simulink model "vehicleHVAC"  (R2016a)
settings: Solver=VariableStepAuto  SolverMode=SingleTasking  StartTime=0.0  StopTime=2000  RelTol=1e-3
PreLoadFcn:
  | T_init = 25; % degC
  | RH_init = 0.5;
  | p_env = 101.325; % kPa
  | 
  | T_coolant = 90; % degC
  | C_coolant = 0.7; % kW/K
  | T_refrigerant = 4; % degC
  | 
  | cabin_volume = 3; % m^3
  | duct_area = 0.015; % m^2
StartFcn:
  | if strcmp(get_param([bdroot, '/System Inputs'], 'OverrideUsingVariant'), 'Manual')
  | 
  |     if exist('h1_vehicleHVAC', 'var') && isgraphics(h1_vehicleHVAC, 'figure')
  |         h1_vehicleHVAC.prepManualInput()
  |     end
  | 
  |     clear updatePsychrometricChart
  |     listener_vehicleHVAC = add_exec_event_listener( ...
  |         [bdroot '/Cabin/Cabin Sensors/Cabin Outputs'], ...
  |         'PostOutputs', ...
  |         @updatePsychrometricChart);
  | 
  | else
  | 
  |     clear listener_vehicleHVAC
  | 
  | end
StopFcn:
  | clear listener_vehicleHVAC
undefined symbols (not defined in the file or in its folder): sigbuilder_block
libraries: fl_lib x26, nesl_utility x22, HVAC_lib x16
CloseFcn:
  | try, close(h1_vehicleHVAC), end
  | clear h1_vehicleHVAC
  | 
  | clear simlog_vehicleHVAC tout
  | clear T_init RH_init p_env T_coolant C_coolant T_refrigerant cabin_volume duct_area
Description:
  | Vehicle HVAC System
  | 
  | Copyright 2017 The MathWorks, Inc.
settings Model: Creator=leong  LastModifiedBy=leong
settings SolverCC: MaxConsecutiveMinStep=2
settings DataIOCC: LimitDataPoints=on  MaxDataPoints=10000
settings DebuggingCC: SFUnexpectedBacktrackingDiag=error  SFNoUnconditionalDefaultTransitionDiag=error
settings GRTTargetCC: TargetLangStandard=C99 (ISO)  GeneratePreprocessorConditionals=Use local settings
settings ConfigComp: CovMetricSettings=dwe  CovHtmlReporting=off  CovSaveCumulativeToWorkspaceVar=off  CovSaveSingleToWorkspaceVar=off  CovExternalEMLEnable=on
settings SimscapeCC: SimscapeLogType=all  SimscapeLogSimulationStatistics=on  SimscapeLogName=simlog_vehicleHVAC  SimscapeLogDataHistory=10000

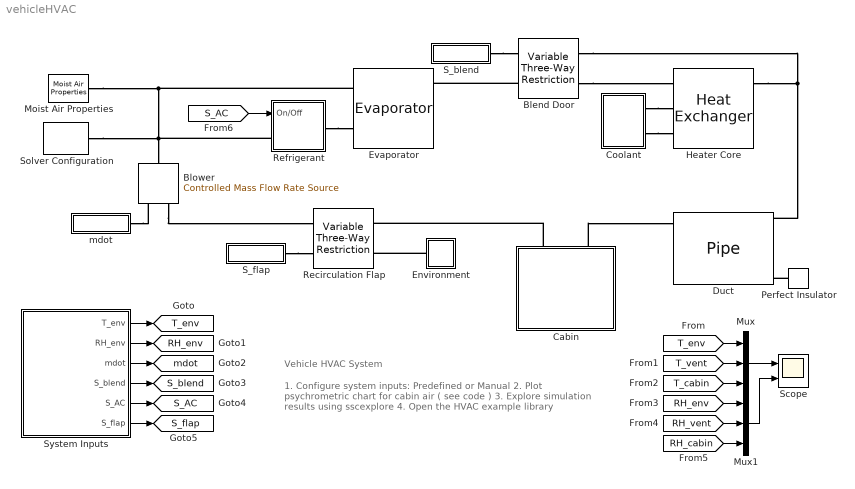
== system vehicleHVAC ==
  note: Vehicle HVAC System
  note: 1. Configure system inputs: Predefined or Manual
      | 2. Plot psychrometric chart for cabin air ( see code )
      | 3. Explore simulation results using sscexplore
      | 4. Open the HVAC example library
  Blend Door : HVAC_lib/Variable Three-Way Restriction  min_area=1e-10 m^2  max_area=0.9 * duct_area m^2  area=duct_area m^2  Cd=0.8  B_lam=0.999
  Blower : HVAC_lib/Controlled Mass Flow Rate Source  flow_area_A=0.01 m^2  flow_area_B=0.01 m^2  area_A=duct_area m^2  area_B=duct_area m^2  mdot_A_specify=off  mdot_A_priority=None  mdot_A=1e-6 kg/s  mdot_B_specify=off  mdot_B_priority=None  mdot_B=1e-6 kg/s  Phi_A_specify=off  Phi_A_priority=None  Phi_A=0 kW  Phi_B_specify=off  Phi_B_priority=None  Phi_B=0 kW  mdot_w_A_specify=off  mdot_w_A_priority=None  mdot_w_A=0 g/s  mdot_w_B_specify=off  mdot_w_B_priority=None  mdot_w_B=0 g/s  h_out_specify=off  h_out_priority=None  h_out=420 kJ/kg  x_w_out_specify=off  x_w_out_priority=None  x_w_out=0.007  power_specify=off  power_priority=None  power=0 kW
  Cabin : Subsystem  Tag=PublishSubsystem  mask{N_occupant=1, W_occupant=0.04, T_occupant=30, Q_occupant=70}
      mask prompts: N_occupant "Number of occupants"; W_occupant "Moisture gain per occupant (g/s)"; T_occupant "Temperature of added moisture (degC)"; Q_occupant "Sensible heat per occupant (W)"
  Coolant : Subsystem
  Duct : HVAC_lib/Pipe  flow_area_A=0.01 m^2  flow_area_B=0.01 m^2  length=1 m  area=duct_area m^2  Dh=sqrt(duct_area) m  length_add=0 m  roughness=15e-6 m  Re_lam=2000  Re_tur=4000  shape_factor=64  Nu_lam=3.66  time_constant=1e-3 s  mdot_A_specify=off  mdot_A_priority=None  mdot_A=1e-6 kg/s  mdot_B_specify=off  mdot_B_priority=None  mdot_B=1e-6 kg/s  Phi_A_specify=off  Phi_A_priority=None  Phi_A=0 kW  Phi_B_specify=off  Phi_B_priority=None  Phi_B=0 kW  mdot_w_A_specify=off  mdot_w_A_priority=None  mdot_w_A=0 g/s  mdot_w_B_specify=off  mdot_w_B_priority=None  mdot_w_B=0 g/s  h_out_specify=off  h_out_priority=None  h_out=420 kJ/kg  x_w_out_specify=off  x_w_out_priority=None  x_w_out=0.007  p_I_specify=on  p_I_priority=High  p_I=p_env kPa  T_I_specify=on  T_I_priority=High  T_I=T_init degC  RH_I_specify=on  RH_I_priority=High  RH_I=RH_init  Q_H_specify=off  Q_H_priority=None  Q_H=0 kW  rho_I_specify=off  rho_I_priority=None  rho_I=1.2 kg/m^3  x_w_sat_specify=off  x_w_sat_priority=None  x_w_sat=0.01  log_p_w_sat_specify=off  log_p_w_sat_priority=None  log_p_w_sat=8  pressure_loss_A_specify=off  pressure_loss_A_priority=None  pressure_loss_A=0 kPa  pressure_loss_B_specify=off  pressure_loss_B_priority=None  pressure_loss_B=0 kPa
  Environment : Subsystem
  Evaporator : HVAC_lib/Evaporator  flow_area_A=0.01 m^2  flow_area_B=0.01 m^2  UA=0.4 kW/K  loss_coeff=2  volume=2e-3 m^3  port_area=duct_area m^2  time_constant=1e-3 s  mdot_A_specify=off  mdot_A_priority=None  mdot_A=1e-6 kg/s  mdot_B_specify=off  mdot_B_priority=None  mdot_B=1e-6 kg/s  Phi_A_specify=off  Phi_A_priority=None  Phi_A=0 kW  Phi_B_specify=off  Phi_B_priority=None  Phi_B=0 kW  mdot_w_A_specify=off  mdot_w_A_priority=None  mdot_w_A=0 g/s  mdot_w_B_specify=off  mdot_w_B_priority=None  mdot_w_B=0 g/s  h_out_specify=off  h_out_priority=None  h_out=420 kJ/kg  x_w_out_specify=off  x_w_out_priority=None  x_w_out=0.007  p_I_specify=on  p_I_priority=High  p_I=p_env kPa  T_I_specify=on  T_I_priority=High  T_I=T_init degC  RH_I_specify=on  RH_I_priority=High  RH_I=RH_init  Q_hex_specify=off  Q_hex_priority=None  Q_hex=0 kW  rho_I_specify=off  rho_I_priority=None  rho_I=1.2 kg/m^3  x_w_sat_specify=off  x_w_sat_priority=None  x_w_sat=0.01  log_p_w_sat_specify=off  log_p_w_sat_priority=None  log_p_w_sat=8  C_min_specify=off  C_min_priority=None  C_min=1 kW/K  effectiveness_specify=off  effectiveness_priority=None  effectiveness=1
  Heater Core : HVAC_lib/Heat Exchanger  flow_area_A=0.01 m^2  flow_area_B=0.01 m^2  UA=0.4 kW/K  loss_coeff=2  volume=1e-3 m^3  port_area=duct_area m^2  time_constant=1e-3 s  mdot_A_specify=off  mdot_A_priority=None  mdot_A=1e-6 kg/s  mdot_B_specify=off  mdot_B_priority=None  mdot_B=1e-6 kg/s  Phi_A_specify=off  Phi_A_priority=None  Phi_A=0 kW  Phi_B_specify=off  Phi_B_priority=None  Phi_B=0 kW  mdot_w_A_specify=off  mdot_w_A_priority=None  mdot_w_A=0 g/s  mdot_w_B_specify=off  mdot_w_B_priority=None  mdot_w_B=0 g/s  h_out_specify=off  h_out_priority=None  h_out=420 kJ/kg  x_w_out_specify=off  x_w_out_priority=None  x_w_out=0.007  p_I_specify=on  p_I_priority=High  p_I=p_env kPa  T_I_specify=on  T_I_priority=High  T_I=T_init degC  RH_I_specify=on  RH_I_priority=High  RH_I=RH_init  Q_hex_specify=off  Q_hex_priority=None  Q_hex=0 kW  rho_I_specify=off  rho_I_priority=None  rho_I=1.2 kg/m^3  x_w_sat_specify=off  x_w_sat_priority=None  x_w_sat=0.01  log_p_w_sat_specify=off  log_p_w_sat_priority=None  log_p_w_sat=8  C_min_specify=off  C_min_priority=None  C_min=1 kW/K  C_max_specify=off  C_max_priority=None  C_max=1 kW/K  effectiveness_specify=off  effectiveness_priority=None  effectiveness=1
  Moist Air Properties : HVAC_lib/Moist Air Properties  MM_da=28.96546 g/mol  MM_w=18.015268 g/mol  Ru=8.3144598 J/K/mol  mu_ref=18 s*uPa  k_ref=26 mW/m/K  D_ref=25 mm^2/s  p_w_sat_coeff=[-5800.2206; 1.3914993; -0.048640239; 4.1764768e-5; -1.4452093e-8; 6.5459673]  T_ref=20 degC  h_da_ref=20.12 kJ/kg  h_w_ref=2538.2 kJ/kg  h_l_ref=83.72 kJ/kg  cp_da_ref=1.006 kJ/kg/K  cp_w_ref=1.86 kJ/kg/K  cp_l_ref=4.186 kJ/kg/K  p_min=1 kPa  p_max=100 MPa  T_min=0 degC  T_max=200 degC
  Mux : Mux  Inputs=3
  Mux1 : Mux  Inputs=3
  Perfect Insulator : fl_lib/Thermal/Thermal Elements/Perfect Insulator  T_specify=off  T_priority=None  T=0 K
  Recirculation Flap : HVAC_lib/Variable Three-Way Restriction  min_area=1e-10 m^2  max_area=0.9 * duct_area m^2  area=duct_area m^2  Cd=0.8  B_lam=0.999
  Refrigerant : Subsystem
  S_blend : Subsystem
      mask Display: disp(get_param(gcb, 'Name'))
  S_flap : Subsystem
      mask Display: disp(get_param(gcb, 'Name'))
  Scope : Scope  NumInputPorts=2
  Solver Configuration : nesl_utility/Solver Configuration  PhysicalDomain=network_engine_domain  SubClassName=solver  LeftPortType=input  RightPortType=generic  Accelerate=off  Tones=[]  Harmonics=[]  SimulateNoise=off  Profile=off  UseLocalSampling=off  EnableSwitchedLinearOptims=on  FrequencyDomain=off  UseCCode=off  RelTol=0.001  AbsTol=1e-06  MinStep=1e-09  ToWorkspace=off  RevertToSquareIcSolve=off  NumHomotopyIterations=100  PhasorMode=off  PhasorModeNumHarmonics=1  OverrideAbsTol=off  DoDC=off  ResidualTolerance=1e-9  UseLocalSolver=off  LocalSolverChoice=NE_BACKWARD_EULER_ADVANCER  LocalSolverSampleTime=0.01  DoFixedCost=off  MaxNonlinIter=3  MaxModeIter=2  LinearAlgebra=Sparse  DelaysMemoryBudget=1024  AutomaticFiltering=on  FilteringTimeConstant=0.001
  System Inputs : Subsystem  Variant=on  VariantControl=Variant1  OverrideUsingVariant=Predefined
      settings: AttributesFormatString=%<ActiveVariant>
  mdot : Subsystem
      mask Display: disp(get_param(gcb, 'Name'))
  tag scope: RH_env=global, S_AC=global, S_blend=global, S_flap=global, T_env=global, mdot=global
  wires:
  [S_AC] -> Refrigerant/1(On/Off)
  [T_cabin] -> Mux/3
  [T_vent] -> Mux/2
  [T_env] -> Mux/1
  [RH_env] -> Mux1/1
  [RH_vent] -> Mux1/2
  [RH_cabin] -> Mux1/3
  Mux/1 -> Scope/1
  Mux1/1 -> Scope/2
  System Inputs/1(" T_env") -> [T_env]
  System Inputs/2(" RH_env") -> [RH_env]
  System Inputs/3(" mdot") -> [mdot]
  System Inputs/4(" S_blend") -> [S_blend]
  System Inputs/5(S_AC) -> [S_AC]
  System Inputs/6(" S_flap") -> [S_flap]
  connections:
  Cabin/LConn2 -- Duct/RConn1
  Cabin/LConn1 -- Recirculation Flap/RConn1
  Blower/LConn1 -- Recirculation Flap/LConn1
  Evaporator/LConn1 -- Moist Air Properties/RConn1 -- Solver Configuration/RConn1 -- Refrigerant/LConn1 -- Blower/RConn1
  Blend Door/LConn1 -- Evaporator/RConn1
  Blend Door/RConn1 -- Heater Core/LConn1
  Heater Core/RConn1 -- Duct/LConn1 -- Blend Door/RConn2
  Perfect Insulator/LConn1 -- Duct/LConn4
  Refrigerant/RConn1 -- Evaporator/LConn2
  S_flap/RConn1 -- Recirculation Flap/LConn2
  S_blend/RConn1 -- Blend Door/LConn2
  mdot/RConn1 -- Blower/LConn2
  Coolant/RConn1 -- Heater Core/LConn2
  Coolant/RConn2 -- Heater Core/LConn3
  Environment/LConn1 -- Recirculation Flap/RConn2

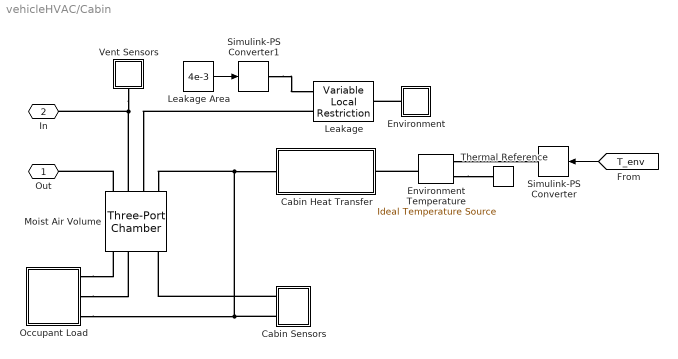
== system vehicleHVAC/Cabin ==
  Cabin Heat Transfer : Subsystem  Tag=PublishSubsystem
  Cabin Sensors : Subsystem
  Environment : Subsystem
  Environment Temperature : fl_lib/Thermal/Thermal Sources/Ideal Temperature Source
  Leakage : HVAC_lib/Variable Local Restriction  flow_area_A=0.01 m^2  flow_area_B=0.01 m^2  min_area=1e-10 m^2  max_area=0.9 m^2  area=1 m^2  Cd=0.8  B_lam=0.999  mdot_A_specify=off  mdot_A_priority=None  mdot_A=1e-6 kg/s  mdot_B_specify=off  mdot_B_priority=None  mdot_B=1e-6 kg/s  Phi_A_specify=off  Phi_A_priority=None  Phi_A=0 kW  Phi_B_specify=off  Phi_B_priority=None  Phi_B=0 kW  mdot_w_A_specify=off  mdot_w_A_priority=None  mdot_w_A=0 g/s  mdot_w_B_specify=off  mdot_w_B_priority=None  mdot_w_B=0 g/s  h_out_specify=off  h_out_priority=None  h_out=420 kJ/kg  x_w_out_specify=off  x_w_out_priority=None  x_w_out=0.007  rho_avg_specify=off  rho_avg_priority=None  rho_avg=1.2 kg/m^3
  Leakage Area : Constant  Value=4e-3
  Moist Air Volume : HVAC_lib/Three-Port Chamber  flow_area_A=0.01 m^2  flow_area_B=0.01 m^2  flow_area_C=0.01 m^2  volume=cabin_volume m^3  area_A=duct_area m^2  area_B=duct_area m^2  area_C=1 m^2  time_constant=1e-3 s  mdot_A_specify=off  mdot_A_priority=None  mdot_A=1e-6 kg/s  mdot_B_specify=off  mdot_B_priority=None  mdot_B=1e-6 kg/s  mdot_C_specify=off  mdot_C_priority=None  mdot_C=1e-6 kg/s  Phi_A_specify=off  Phi_A_priority=None  Phi_A=0 kW  Phi_B_specify=off  Phi_B_priority=None  Phi_B=0 kW  Phi_C_specify=off  Phi_C_priority=None  Phi_C=0 kW  mdot_w_A_specify=off  mdot_w_A_priority=None  mdot_w_A=0 g/s  mdot_w_B_specify=off  mdot_w_B_priority=None  mdot_w_B=0 g/s  mdot_w_C_specify=off  mdot_w_C_priority=None  mdot_w_C=0 g/s  h_out_specify=off  h_out_priority=None  h_out=420 kJ/kg  x_w_out_specify=off  x_w_out_priority=None  x_w_out=0.007  p_I_specify=on  p_I_priority=High  p_I=p_env kPa  T_I_specify=on  T_I_priority=High  T_I=T_init degC  RH_I_specify=on  RH_I_priority=High  RH_I=RH_init  Q_H_specify=off  Q_H_priority=None  Q_H=0 kW  rho_I_specify=off  rho_I_priority=None  rho_I=1.2 kg/m^3  x_w_sat_specify=off  x_w_sat_priority=None  x_w_sat=0.01  log_p_w_sat_specify=off  log_p_w_sat_priority=None  log_p_w_sat=8
  Occupant Load : Subsystem
  Simulink-PS Converter : nesl_utility/Simulink-PS Converter  PhysicalDomain=network_engine_domain  SubClassName=ps_input  LeftPortType=input  RightPortType=output  PseudoPeriodic=off  Frequencies=[]  NoiseDistribution=none  NoiseParameters=[]  Unit=degC  AffineConversion=on  InputFiltering=off  SimscapeFilterOrder=1  InputFilterTimeConstant=0.001  UdotUserProvided=0
  Simulink-PS Converter1 : nesl_utility/Simulink-PS Converter  PhysicalDomain=network_engine_domain  SubClassName=ps_input  LeftPortType=input  RightPortType=output  PseudoPeriodic=off  Frequencies=[]  NoiseDistribution=none  NoiseParameters=[]  Unit=m^2  AffineConversion=off  InputFiltering=off  SimscapeFilterOrder=1  InputFilterTimeConstant=0.001  UdotUserProvided=0
  Thermal Reference : fl_lib/Thermal/Thermal Elements/Thermal Reference
  Vent Sensors : Subsystem
  Out : PMIOPort  Port=1  Side=Left
  In : PMIOPort  Port=2  Side=Left
  wires:
  Leakage Area/1 -> Simulink-PS Converter1/1
  [T_env] -> Simulink-PS Converter/1
  connections:
  Moist Air Volume/LConn1 -- Out/RConn1
  Environment/LConn1 -- Leakage/RConn1
  Leakage/LConn1 -- Moist Air Volume/LConn3
  Moist Air Volume/LConn2 -- Vent Sensors/LConn1 -- In/RConn1
  Environment Temperature/RConn1 -- Simulink-PS Converter/RConn1
  Occupant Load/RConn3 -- Cabin Sensors/LConn2 -- Cabin Heat Transfer/LConn1 -- Moist Air Volume/LConn4
  Environment Temperature/LConn1 -- Cabin Heat Transfer/RConn1
  Cabin Sensors/LConn1 -- Moist Air Volume/RConn4
  Environment Temperature/RConn2 -- Thermal Reference/LConn1
  Simulink-PS Converter1/RConn1 -- Leakage/LConn2
  Occupant Load/RConn1 -- Moist Air Volume/RConn1
  Occupant Load/RConn2 -- Moist Air Volume/RConn2

== system vehicleHVAC/Coolant ==
  Coolant Capacity Rate : Constant  Value=C_coolant
  Coolant Temperature : Constant  Value=T_coolant
  Simulink-PS Converter : nesl_utility/Simulink-PS Converter  PhysicalDomain=network_engine_domain  SubClassName=ps_input  LeftPortType=input  RightPortType=output  PseudoPeriodic=off  Frequencies=[]  NoiseDistribution=none  NoiseParameters=[]  Unit=degC  AffineConversion=on  InputFiltering=off  SimscapeFilterOrder=1  InputFilterTimeConstant=0.001  UdotUserProvided=0
  Simulink-PS Converter1 : nesl_utility/Simulink-PS Converter  PhysicalDomain=network_engine_domain  SubClassName=ps_input  LeftPortType=input  RightPortType=output  PseudoPeriodic=off  Frequencies=[]  NoiseDistribution=none  NoiseParameters=[]  Unit=kW/K  AffineConversion=off  InputFiltering=off  SimscapeFilterOrder=1  InputFilterTimeConstant=0.001  UdotUserProvided=0
  T2 : PMIOPort  Port=1  Side=Right
  C2 : PMIOPort  Port=2  Side=Right
  wires:
  Coolant Capacity Rate/1 -> Simulink-PS Converter1/1
  Coolant Temperature/1 -> Simulink-PS Converter/1
  connections:
  Simulink-PS Converter1/RConn1 -- C2/RConn1
  Simulink-PS Converter/RConn1 -- T2/RConn1

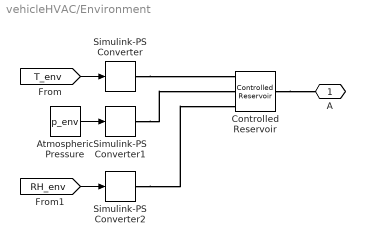
== system vehicleHVAC/Environment ==
  Atmospheric Pressure : Constant  Value=p_env
  Controlled Reservoir : HVAC_lib/Controlled Reservoir  flow_area_A=0.01 m^2  area_A=duct_area m^2  mdot_A_specify=off  mdot_A_priority=None  mdot_A=1e-6 kg/s  Phi_A_specify=off  Phi_A_priority=None  Phi_A=0 kW  mdot_w_A_specify=off  mdot_w_A_priority=None  mdot_w_A=0 g/s  h_out_specify=off  h_out_priority=None  h_out=420 kJ/kg  x_w_out_specify=off  x_w_out_priority=None  x_w_out=0.007  log_p_w_sat_specify=off  log_p_w_sat_priority=None  log_p_w_sat=8
  Simulink-PS Converter : nesl_utility/Simulink-PS Converter  PhysicalDomain=network_engine_domain  SubClassName=ps_input  LeftPortType=input  RightPortType=output  PseudoPeriodic=off  Frequencies=[]  NoiseDistribution=none  NoiseParameters=[]  Unit=degC  AffineConversion=on  InputFiltering=off  SimscapeFilterOrder=1  InputFilterTimeConstant=0.001  UdotUserProvided=0
  Simulink-PS Converter1 : nesl_utility/Simulink-PS Converter  PhysicalDomain=network_engine_domain  SubClassName=ps_input  LeftPortType=input  RightPortType=output  PseudoPeriodic=off  Frequencies=[]  NoiseDistribution=none  NoiseParameters=[]  Unit=kPa  AffineConversion=off  InputFiltering=off  SimscapeFilterOrder=1  InputFilterTimeConstant=0.001  UdotUserProvided=0
  Simulink-PS Converter2 : nesl_utility/Simulink-PS Converter  PhysicalDomain=network_engine_domain  SubClassName=ps_input  LeftPortType=input  RightPortType=output  PseudoPeriodic=off  Frequencies=[]  NoiseDistribution=none  NoiseParameters=[]  Unit=1  AffineConversion=off  InputFiltering=off  SimscapeFilterOrder=1  InputFilterTimeConstant=0.001  UdotUserProvided=0
  A : PMIOPort  Port=1  Side=Left
  wires:
  Atmospheric Pressure/1 -> Simulink-PS Converter1/1
  [RH_env] -> Simulink-PS Converter2/1
  [T_env] -> Simulink-PS Converter/1
  connections:
  Controlled Reservoir/LConn1 -- A/RConn1
  Simulink-PS Converter/RConn1 -- Controlled Reservoir/RConn1
  Simulink-PS Converter1/RConn1 -- Controlled Reservoir/RConn2
  Simulink-PS Converter2/RConn1 -- Controlled Reservoir/RConn3

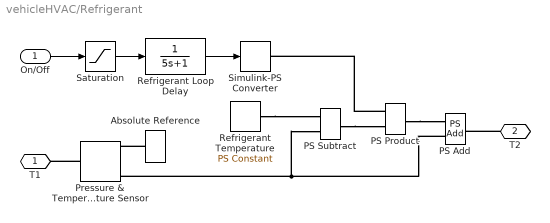
== system vehicleHVAC/Refrigerant ==
  On/Off : Inport
  Absolute Reference : HVAC_lib/Absolute Reference  mdot_specify=off  mdot_priority=None  mdot=1e-6 kg/s  Phi_specify=off  Phi_priority=None  Phi=0 kW  mdot_w_specify=off  mdot_w_priority=None  mdot_w=0 kg/s
  PS Add : fl_lib/Physical Signals/Functions/PS Add
  PS Product : fl_lib/Physical Signals/Functions/PS Product
  PS Subtract : fl_lib/Physical Signals/Functions/PS Subtract
  Pressure & Temperature Sensor : HVAC_lib/Pressure & Temperature Sensor
  Refrigerant Loop Delay : TransferFcn  Denominator=[5 1]
  Refrigerant Temperature : fl_lib/Physical Signals/Sources/PS Constant  constant=T_refrigerant + 273.15
  Saturation : Saturate  UpperLimit=1  LowerLimit=0  ZeroCross=off
  Simulink-PS Converter : nesl_utility/Simulink-PS Converter  PhysicalDomain=network_engine_domain  SubClassName=ps_input  LeftPortType=input  RightPortType=output  PseudoPeriodic=off  Frequencies=[]  NoiseDistribution=none  NoiseParameters=[]  Unit=1  AffineConversion=off  InputFiltering=off  SimscapeFilterOrder=1  InputFilterTimeConstant=0.001  UdotUserProvided=0
  T1 : PMIOPort  Port=1  Side=Left
  T2 : PMIOPort  Port=2  Side=Right
  wires:
  On/Off/1 -> Saturation/1
  Saturation/1 -> Refrigerant Loop Delay/1
  Refrigerant Loop Delay/1 -> Simulink-PS Converter/1
  connections:
  Absolute Reference/LConn1 -- Pressure & Temperature Sensor/RConn1
  Pressure & Temperature Sensor/LConn1 -- T1/RConn1
  PS Add/LConn2 -- PS Subtract/LConn2 -- Pressure & Temperature Sensor/RConn3
  Refrigerant Temperature/RConn1 -- PS Subtract/LConn1
  PS Subtract/RConn1 -- PS Product/LConn2
  PS Product/RConn1 -- PS Add/LConn1
  PS Product/LConn1 -- Simulink-PS Converter/RConn1
  T2/RConn1 -- PS Add/RConn1

== system vehicleHVAC/S_blend ==
  Door Delay : TransferFcn  Denominator=[2 1]
  Simulink-PS Converter : nesl_utility/Simulink-PS Converter  PhysicalDomain=network_engine_domain  SubClassName=ps_input  LeftPortType=input  RightPortType=output  PseudoPeriodic=off  Frequencies=[]  NoiseDistribution=none  NoiseParameters=[]  Unit=1  AffineConversion=off  InputFiltering=off  SimscapeFilterOrder=1  InputFilterTimeConstant=0.001  UdotUserProvided=0
  S_blend : PMIOPort  Port=1  Side=Right
  wires:
  [S_blend] -> Door Delay/1
  Door Delay/1 -> Simulink-PS Converter/1
  connections:
  Simulink-PS Converter/RConn1 -- S_blend/RConn1

== system vehicleHVAC/S_flap ==
  Flap Delay : TransferFcn  Denominator=[2 1]
  Simulink-PS Converter : nesl_utility/Simulink-PS Converter  PhysicalDomain=network_engine_domain  SubClassName=ps_input  LeftPortType=input  RightPortType=output  PseudoPeriodic=off  Frequencies=[]  NoiseDistribution=none  NoiseParameters=[]  Unit=1  AffineConversion=off  InputFiltering=off  SimscapeFilterOrder=1  InputFilterTimeConstant=0.001  UdotUserProvided=0
  S_flap : PMIOPort  Port=1  Side=Right
  wires:
  Flap Delay/1 -> Simulink-PS Converter/1
  [S_flap] -> Flap Delay/1
  connections:
  Simulink-PS Converter/RConn1 -- S_flap/RConn1

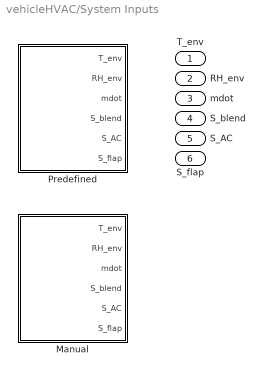
== system vehicleHVAC/System Inputs ==
  Manual : Subsystem  Tag=PublishSubsystem  VariantControl=Manual
  Predefined : Subsystem  VariantControl=Predefined
  " T_env" : Outport
  " RH_env" : Outport  Port=2
  " mdot" : Outport  Port=3
  " S_blend" : Outport  Port=4
  S_AC : Outport  Port=5
  " S_flap" : Outport  Port=6

== system vehicleHVAC/mdot ==
  Blower Delay : TransferFcn  Denominator=[1 1]
  Simulink-PS Converter : nesl_utility/Simulink-PS Converter  PhysicalDomain=network_engine_domain  SubClassName=ps_input  LeftPortType=input  RightPortType=output  PseudoPeriodic=off  Frequencies=[]  NoiseDistribution=none  NoiseParameters=[]  Unit=kg/s  AffineConversion=off  InputFiltering=off  SimscapeFilterOrder=1  InputFilterTimeConstant=0.001  UdotUserProvided=0
  mdot : PMIOPort  Port=1  Side=Right
  wires:
  Blower Delay/1 -> Simulink-PS Converter/1
  [mdot] -> Blower Delay/1
  connections:
  Simulink-PS Converter/RConn1 -- mdot/RConn1

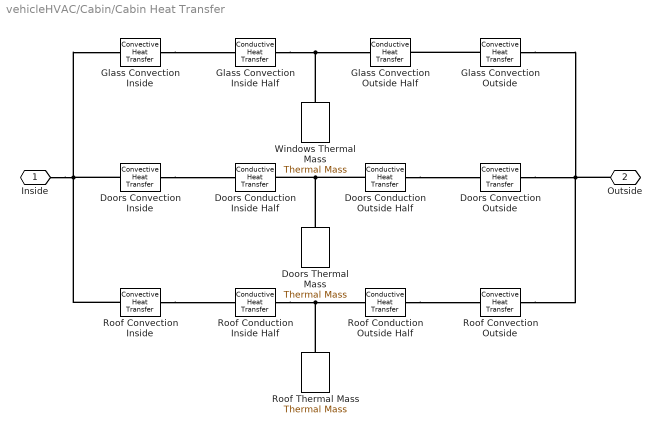
== system vehicleHVAC/Cabin/Cabin Heat Transfer ==
  Doors Thermal Mass : fl_lib/Thermal/Thermal Elements/Thermal Mass  mass=75 kg  sp_heat=500 J/kg/K  T_specify=on  T_priority=High  T=T_init degC  Q_specify=off  Q_priority=None  Q=0 W
  Doors Conduction Inside Half : fl_lib/Thermal/Thermal Elements/Conductive Heat Transfer  area=4 m^2  thickness=0.06 / 2 m  th_cond=0.08 W/(m*K)  Q_specify=off  Q_priority=None  Q=0 W  T_specify=off  T_priority=None  T=0 K
  Doors Conduction Outside Half : fl_lib/Thermal/Thermal Elements/Conductive Heat Transfer  area=4 m^2  thickness=0.06 / 2 m  th_cond=0.08 W/(m*K)  Q_specify=off  Q_priority=None  Q=0 W  T_specify=off  T_priority=None  T=0 K
  Doors Convection Inside : fl_lib/Thermal/Thermal Elements/Convective Heat Transfer  area=4 m^2  heat_tr_coeff=40 W/(m^2 * K)  Q_specify=off  Q_priority=None  Q=0 W  T_specify=off  T_priority=None  T=0 K
  Doors Convection Outside : fl_lib/Thermal/Thermal Elements/Convective Heat Transfer  area=4 m^2  heat_tr_coeff=40 W/(m^2 * K)  Q_specify=off  Q_priority=None  Q=0 W  T_specify=off  T_priority=None  T=0 K
  Glass Convection Inside : fl_lib/Thermal/Thermal Elements/Convective Heat Transfer  area=3.5 m^2  heat_tr_coeff=40 W/(m^2 * K)  Q_specify=off  Q_priority=None  Q=0 W  T_specify=off  T_priority=None  T=0 K
  Glass Convection Inside Half : fl_lib/Thermal/Thermal Elements/Conductive Heat Transfer  area=3.5 m^2  thickness=0.004 / 2 m  th_cond=0.96 W/(m*K)  Q_specify=off  Q_priority=None  Q=0 W  T_specify=off  T_priority=None  T=0 K
  Glass Convection Outside : fl_lib/Thermal/Thermal Elements/Convective Heat Transfer  area=3.5 m^2  heat_tr_coeff=40 W/(m^2 * K)  Q_specify=off  Q_priority=None  Q=0 W  T_specify=off  T_priority=None  T=0 K
  Glass Convection Outside Half : fl_lib/Thermal/Thermal Elements/Conductive Heat Transfer  area=3.5 m^2  thickness=0.004 / 2 m  th_cond=0.96 W/(m*K)  Q_specify=off  Q_priority=None  Q=0 W  T_specify=off  T_priority=None  T=0 K
  Roof Thermal Mass : fl_lib/Thermal/Thermal Elements/Thermal Mass  mass=30 kg  sp_heat=500 J/kg/K  T_specify=on  T_priority=High  T=T_init degC  Q_specify=off  Q_priority=None  Q=0 W
  Roof Conduction Inside Half : fl_lib/Thermal/Thermal Elements/Conductive Heat Transfer  area=2 m^2  thickness=0.04 / 2 m  th_cond=0.08 W/(m*K)  Q_specify=off  Q_priority=None  Q=0 W  T_specify=off  T_priority=None  T=0 K
  Roof Conduction Outside Half : fl_lib/Thermal/Thermal Elements/Conductive Heat Transfer  area=2 m^2  thickness=0.04 / 2 m  th_cond=0.08 W/(m*K)  Q_specify=off  Q_priority=None  Q=0 W  T_specify=off  T_priority=None  T=0 K
  Roof Convection Inside : fl_lib/Thermal/Thermal Elements/Convective Heat Transfer  area=2 m^2  heat_tr_coeff=40 W/(m^2 * K)  Q_specify=off  Q_priority=None  Q=0 W  T_specify=off  T_priority=None  T=0 K
  Roof Convection Outside : fl_lib/Thermal/Thermal Elements/Convective Heat Transfer  area=2 m^2  heat_tr_coeff=40 W/(m^2 * K)  Q_specify=off  Q_priority=None  Q=0 W  T_specify=off  T_priority=None  T=0 K
  Windows Thermal Mass : fl_lib/Thermal/Thermal Elements/Thermal Mass  mass=3.5 * 0.004 * 2600 kg  sp_heat=840 J/kg/K  T_specify=on  T_priority=High  T=T_init degC  Q_specify=off  Q_priority=None  Q=0 W
  Inside : PMIOPort  Port=1  Side=Left
  Outside : PMIOPort  Port=2  Side=Right
  connections:
  Glass Convection Inside/RConn1 -- Glass Convection Inside Half/LConn1
  Glass Convection Outside/LConn1 -- Glass Convection Outside Half/RConn1
  Doors Conduction Outside Half/RConn1 -- Doors Convection Outside/LConn1
  Roof Conduction Outside Half/RConn1 -- Roof Convection Outside/LConn1
  Roof Conduction Inside Half/RConn1 -- Roof Thermal Mass/LConn1 -- Roof Conduction Outside Half/LConn1
  Glass Convection Inside Half/RConn1 -- Windows Thermal Mass/LConn1 -- Glass Convection Outside Half/LConn1
  Doors Convection Inside/RConn1 -- Doors Conduction Inside Half/LConn1
  Doors Convection Outside/RConn1 -- Outside/RConn1 -- Glass Convection Outside/RConn1 -- Roof Convection Outside/RConn1
  Doors Conduction Outside Half/LConn1 -- Doors Thermal Mass/LConn1 -- Doors Conduction Inside Half/RConn1
  Roof Convection Inside/RConn1 -- Roof Conduction Inside Half/LConn1
  Inside/RConn1 -- Glass Convection Inside/LConn1 -- Doors Convection Inside/LConn1 -- Roof Convection Inside/LConn1

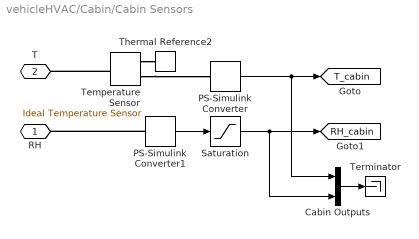
== system vehicleHVAC/Cabin/Cabin Sensors ==
  Cabin Outputs : Concatenate
  PS-Simulink Converter : nesl_utility/PS-Simulink Converter  PhysicalDomain=network_engine_domain  SubClassName=ps_output  LeftPortType=input  RightPortType=output  PseudoPeriodic=off  Frequencies=[]  Unit=degC  AffineConversion=on
  PS-Simulink Converter1 : nesl_utility/PS-Simulink Converter  PhysicalDomain=network_engine_domain  SubClassName=ps_output  LeftPortType=input  RightPortType=output  PseudoPeriodic=off  Frequencies=[]  Unit=1  AffineConversion=off
  Saturation : Saturate  UpperLimit=1  LowerLimit=0  ZeroCross=off
  Temperature Sensor : fl_lib/Thermal/Thermal Sensors/Ideal Temperature Sensor
  Terminator : Terminator
  Thermal Reference2 : fl_lib/Thermal/Thermal Elements/Thermal Reference
  RH : PMIOPort  Port=1  Side=Left
  T : PMIOPort  Port=2  Side=Left
  tag scope: RH_cabin=global, T_cabin=global
  wires:
  PS-Simulink Converter/1 -> Cabin Outputs/1, [T_cabin]
  PS-Simulink Converter1/1 -> Saturation/1
  Cabin Outputs/1 -> Terminator/1
  Saturation/1 -> Cabin Outputs/2, [RH_cabin]
  connections:
  Temperature Sensor/LConn1 -- T/RConn1
  PS-Simulink Converter1/LConn1 -- RH/RConn1
  Temperature Sensor/RConn2 -- PS-Simulink Converter/LConn1
  Temperature Sensor/RConn1 -- Thermal Reference2/LConn1

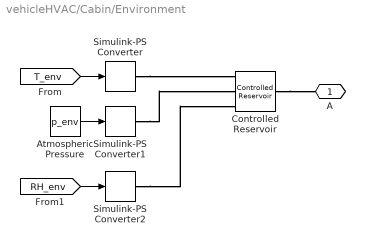
== system vehicleHVAC/Cabin/Environment ==
  Atmospheric Pressure : Constant  Value=p_env
  Controlled Reservoir : HVAC_lib/Controlled Reservoir  flow_area_A=0.01 m^2  area_A=1 m^2  mdot_A_specify=off  mdot_A_priority=None  mdot_A=1e-6 kg/s  Phi_A_specify=off  Phi_A_priority=None  Phi_A=0 kW  mdot_w_A_specify=off  mdot_w_A_priority=None  mdot_w_A=0 g/s  h_out_specify=off  h_out_priority=None  h_out=420 kJ/kg  x_w_out_specify=off  x_w_out_priority=None  x_w_out=0.007  log_p_w_sat_specify=off  log_p_w_sat_priority=None  log_p_w_sat=8
  Simulink-PS Converter : nesl_utility/Simulink-PS Converter  PhysicalDomain=network_engine_domain  SubClassName=ps_input  LeftPortType=input  RightPortType=output  PseudoPeriodic=off  Frequencies=[]  NoiseDistribution=none  NoiseParameters=[]  Unit=degC  AffineConversion=on  InputFiltering=off  SimscapeFilterOrder=1  InputFilterTimeConstant=0.001  UdotUserProvided=0
  Simulink-PS Converter1 : nesl_utility/Simulink-PS Converter  PhysicalDomain=network_engine_domain  SubClassName=ps_input  LeftPortType=input  RightPortType=output  PseudoPeriodic=off  Frequencies=[]  NoiseDistribution=none  NoiseParameters=[]  Unit=kPa  AffineConversion=off  InputFiltering=off  SimscapeFilterOrder=1  InputFilterTimeConstant=0.001  UdotUserProvided=0
  Simulink-PS Converter2 : nesl_utility/Simulink-PS Converter  PhysicalDomain=network_engine_domain  SubClassName=ps_input  LeftPortType=input  RightPortType=output  PseudoPeriodic=off  Frequencies=[]  NoiseDistribution=none  NoiseParameters=[]  Unit=1  AffineConversion=off  InputFiltering=off  SimscapeFilterOrder=1  InputFilterTimeConstant=0.001  UdotUserProvided=0
  A : PMIOPort  Port=1  Side=Left
  wires:
  Atmospheric Pressure/1 -> Simulink-PS Converter1/1
  [RH_env] -> Simulink-PS Converter2/1
  [T_env] -> Simulink-PS Converter/1
  connections:
  Controlled Reservoir/LConn1 -- A/RConn1
  Simulink-PS Converter/RConn1 -- Controlled Reservoir/RConn1
  Simulink-PS Converter1/RConn1 -- Controlled Reservoir/RConn2
  Simulink-PS Converter2/RConn1 -- Controlled Reservoir/RConn3

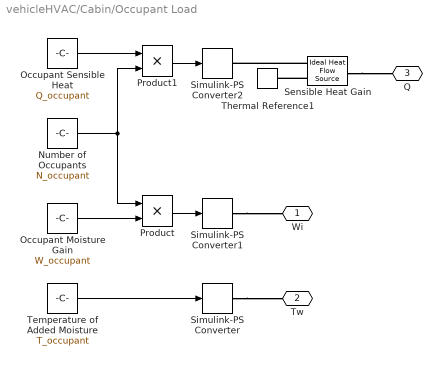
== system vehicleHVAC/Cabin/Occupant Load ==
  Number of Occupants : Constant  Value=N_occupant
  Occupant Moisture Gain : Constant  Value=W_occupant
  Occupant Sensible Heat : Constant  Value=Q_occupant
  Product : Product
  Product1 : Product
  Sensible Heat Gain : fl_lib/Thermal/Thermal Sources/Ideal Heat Flow Source
  Simulink-PS Converter : nesl_utility/Simulink-PS Converter  PhysicalDomain=network_engine_domain  SubClassName=ps_input  LeftPortType=input  RightPortType=output  PseudoPeriodic=off  Frequencies=[]  NoiseDistribution=none  NoiseParameters=[]  Unit=degC  AffineConversion=on  InputFiltering=off  SimscapeFilterOrder=1  InputFilterTimeConstant=0.001  UdotUserProvided=0
  Simulink-PS Converter1 : nesl_utility/Simulink-PS Converter  PhysicalDomain=network_engine_domain  SubClassName=ps_input  LeftPortType=input  RightPortType=output  PseudoPeriodic=off  Frequencies=[]  NoiseDistribution=none  NoiseParameters=[]  Unit=g/s  AffineConversion=off  InputFiltering=off  SimscapeFilterOrder=1  InputFilterTimeConstant=0.001  UdotUserProvided=0
  Simulink-PS Converter2 : nesl_utility/Simulink-PS Converter  PhysicalDomain=network_engine_domain  SubClassName=ps_input  LeftPortType=input  RightPortType=output  PseudoPeriodic=off  Frequencies=[]  NoiseDistribution=none  NoiseParameters=[]  Unit=W  AffineConversion=off  InputFiltering=off  SimscapeFilterOrder=1  InputFilterTimeConstant=0.001  UdotUserProvided=0
  Temperature of Added Moisture : Constant  Value=T_occupant
  Thermal Reference1 : fl_lib/Thermal/Thermal Elements/Thermal Reference
  Wi : PMIOPort  Port=1  Side=Right
  Tw : PMIOPort  Port=2  Side=Right
  Q : PMIOPort  Port=3  Side=Right
  wires:
  Temperature of Added Moisture/1 -> Simulink-PS Converter/1
  Number of Occupants/1 -> Product/1, Product1/2
  Product/1 -> Simulink-PS Converter1/1
  Product1/1 -> Simulink-PS Converter2/1
  Occupant Sensible Heat/1 -> Product1/1
  Occupant Moisture Gain/1 -> Product/2
  connections:
  Simulink-PS Converter1/RConn1 -- Wi/RConn1
  Simulink-PS Converter/RConn1 -- Tw/RConn1
  Sensible Heat Gain/LConn1 -- Q/RConn1
  Sensible Heat Gain/RConn2 -- Thermal Reference1/LConn1
  Sensible Heat Gain/RConn1 -- Simulink-PS Converter2/RConn1

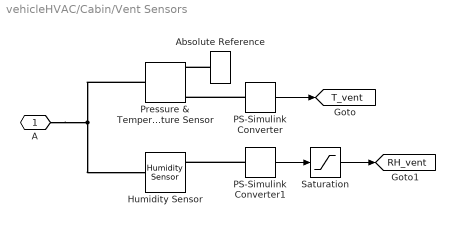
== system vehicleHVAC/Cabin/Vent Sensors ==
  Absolute Reference : HVAC_lib/Absolute Reference  mdot_specify=off  mdot_priority=None  mdot=1e-6 kg/s  Phi_specify=off  Phi_priority=None  Phi=0 kW  mdot_w_specify=off  mdot_w_priority=None  mdot_w=0 kg/s
  Humidity Sensor : HVAC_lib/Humidity Sensor  RH_A_specify=off  RH_A_priority=None  RH_A=0.5  log_p_w_sat_specify=off  log_p_w_sat_priority=None  log_p_w_sat=8
  PS-Simulink Converter : nesl_utility/PS-Simulink Converter  PhysicalDomain=network_engine_domain  SubClassName=ps_output  LeftPortType=input  RightPortType=output  PseudoPeriodic=off  Frequencies=[]  Unit=degC  AffineConversion=on
  PS-Simulink Converter1 : nesl_utility/PS-Simulink Converter  PhysicalDomain=network_engine_domain  SubClassName=ps_output  LeftPortType=input  RightPortType=output  PseudoPeriodic=off  Frequencies=[]  Unit=1  AffineConversion=off
  Pressure & Temperature Sensor : HVAC_lib/Pressure & Temperature Sensor
  Saturation : Saturate  UpperLimit=1  LowerLimit=0  ZeroCross=off
  A : PMIOPort  Port=1  Side=Left
  tag scope: RH_vent=global, T_vent=global
  wires:
  PS-Simulink Converter/1 -> [T_vent]
  PS-Simulink Converter1/1 -> Saturation/1
  Saturation/1 -> [RH_vent]
  connections:
  Pressure & Temperature Sensor/LConn1 -- A/RConn1 -- Humidity Sensor/LConn1
  PS-Simulink Converter/LConn1 -- Pressure & Temperature Sensor/RConn3
  PS-Simulink Converter1/LConn1 -- Humidity Sensor/RConn1
  Absolute Reference/LConn1 -- Pressure & Temperature Sensor/RConn1

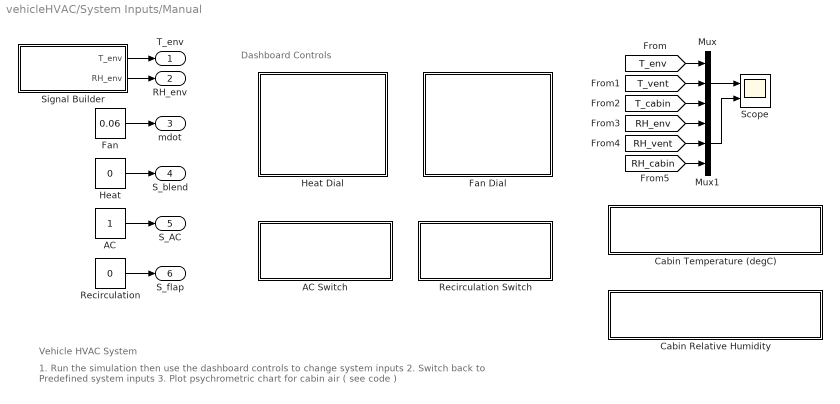
== system vehicleHVAC/System Inputs/Manual ==
  note: Dashboard Controls
  note: 1. Run the simulation then use the dashboard controls to change system inputs
      | 2. Switch back to Predefined system inputs
      | 3. Plot psychrometric chart for cabin air ( see code )
  note: Vehicle HVAC System
  AC : Constant
  AC Switch : Subsystem  DialogController=hmiCreateDDGDialog  IsWebBlock=on  mask(MWDashboardBlock){webBlockId=827ffd02-bfe7-4d14-bd3f-7ef80c0bb8c3, webBlockType=sliderswitch, ShowInLibBrowser=on, ShowInitialText=on, HMISrcModelName=vehicleHVAC}
      mask prompts: webBlockId "WebBlock Id"; webBlockType "WebBlock Type"; HMISrcModelName "Source Model"
      mask help: SimulinkHMI:dialogs:SwitchDialogDesc
      mask Help: helpview([docroot '/mapfiles/simulink.map'], 'hmi_slider_switch')
      mask Display:
      | if strcmp(get_param(bdroot(gcb),'BlockDiagramType'), 'library')
      |     image([(matlabroot) '/toolbox/simulink/hmi/icons/SliderSwitch.png']);
      | end
  Cabin Relative Humidity : Subsystem  DialogController=hmiCreateDDGDialog  IsWebBlock=on  mask(MWDashboardBlock){webBlockId=f2fc8f18-1a55-45da-814e-7c282aae6e84, webBlockType=lineargauge, ShowInLibBrowser=on, ShowInitialText=on, HMISrcModelName=vehicleHVAC}
      mask prompts: webBlockId "WebBlock Id"; webBlockType "WebBlock Type"; HMISrcModelName "Source Model"
      mask help: SimulinkHMI:dialogs:LinearGaugeDialogDesc
      mask Help: helpview([docroot '/mapfiles/simulink.map'], 'hmi_linear_gauge')
      mask Display:
      | if strcmp(get_param(bdroot(gcb),'BlockDiagramType'), 'library')
      |     image([(matlabroot) '/toolbox/simulink/hmi/icons/LinearGauge.png']);
      | end
  Cabin Temperature (degC) : Subsystem  DialogController=hmiCreateDDGDialog  IsWebBlock=on  mask(MWDashboardBlock){webBlockId=20cf081a-ecf9-409a-b722-1806c1b228f7, webBlockType=lineargauge, ShowInLibBrowser=on, ShowInitialText=on, HMISrcModelName=vehicleHVAC}
      mask prompts: webBlockId "WebBlock Id"; webBlockType "WebBlock Type"; HMISrcModelName "Source Model"
      mask help: SimulinkHMI:dialogs:LinearGaugeDialogDesc
      mask Help: helpview([docroot '/mapfiles/simulink.map'], 'hmi_linear_gauge')
      mask Display:
      | if strcmp(get_param(bdroot(gcb),'BlockDiagramType'), 'library')
      |     image([(matlabroot) '/toolbox/simulink/hmi/icons/LinearGauge.png']);
      | end
  Fan : Constant  Value=0.06
  Fan Dial : Subsystem  DialogController=hmiCreateDDGDialog  IsWebBlock=on  mask(MWDashboardBlock){webBlockId=247dfab1-42ee-4734-b4da-45a8d5b10be2, webBlockType=discreteknob, ShowInLibBrowser=on, ShowInitialText=on, HMISrcModelName=vehicleHVAC}
      mask prompts: webBlockId "WebBlock Id"; webBlockType "WebBlock Type"; HMISrcModelName "Source Model"
      mask help: SimulinkHMI:dialogs:DiscreteKnobDialogDesc
      mask Help: helpview([docroot '/mapfiles/simulink.map'], 'hmi_rotary_switch')
      mask Display:
      | model = bdroot(gcb);
      | if strcmp(get_param(model,'BlockDiagramType'), 'library')
      |     image([(matlabroot) '/toolbox/simulink/hmi/icons/DiscreteKnob.png']);
      | end
  Heat : Constant  Value=0
  Heat Dial : Subsystem  DialogController=hmiCreateDDGDialog  IsWebBlock=on  mask(MWDashboardBlock){webBlockId=3ab88035-68a3-4d73-bed1-23b2ea12046f, webBlockType=discreteknob, ShowInLibBrowser=on, ShowInitialText=on, HMISrcModelName=vehicleHVAC}
      mask prompts: webBlockId "WebBlock Id"; webBlockType "WebBlock Type"; HMISrcModelName "Source Model"
      mask help: SimulinkHMI:dialogs:DiscreteKnobDialogDesc
      mask Help: helpview([docroot '/mapfiles/simulink.map'], 'hmi_rotary_switch')
      mask Display:
      | model = bdroot(gcb);
      | if strcmp(get_param(model,'BlockDiagramType'), 'library')
      |     image([(matlabroot) '/toolbox/simulink/hmi/icons/DiscreteKnob.png']);
      | end
  Mux : Mux  Inputs=3
  Mux1 : Mux  Inputs=3
  Recirculation : Constant  Value=0
  Recirculation Switch : Subsystem  DialogController=hmiCreateDDGDialog  IsWebBlock=on  mask(MWDashboardBlock){webBlockId=69c4d9fa-77ef-4507-8636-ae248f6a016c, webBlockType=sliderswitch, ShowInLibBrowser=on, ShowInitialText=on, HMISrcModelName=vehicleHVAC}
      mask prompts: webBlockId "WebBlock Id"; webBlockType "WebBlock Type"; HMISrcModelName "Source Model"
      mask help: SimulinkHMI:dialogs:SwitchDialogDesc
      mask Help: helpview([docroot '/mapfiles/simulink.map'], 'hmi_slider_switch')
      mask Display:
      | if strcmp(get_param(bdroot(gcb),'BlockDiagramType'), 'library')
      |     image([(matlabroot) '/toolbox/simulink/hmi/icons/SliderSwitch.png']);
      | end
  Scope : Scope  NumInputPorts=2
  Signal Builder : Subsystem  Tag=STV Subsys  LoadFcn=sigbuilder_block('load');  StartFcn=sigbuilder_block('start');  StopFcn=sigbuilder_block('stop');  ClipboardFcn=sigbuilder_block('clipboard');  mask(Sigbuilder block){}
      mask help: Simulink:masks:SigbuilderBlock_MD
      mask init:
      | if ~strcmp(get_param(bdroot(gcbh),'SimulationStatus'),'stopped') tuvar = sigbuilder_block('maskInit'); end
      settings: CopyFcn=sigbuilder_block('copy');  DeleteFcn=sigbuilder_block('delete');  ModelCloseFcn=sigbuilder_block('modelClose');  PreSaveFcn=sigbuilder_block('preSave');  PauseFcn=sigbuilder_block('pause');  ContinueFcn=sigbuilder_block('continue');  NameChangeFcn=sigbuilder_block('namechange');  OpenFcn=sigbuilder_block('open',[182.25 533.25 550.5 287.25 ]);  CloseFcn=sigbuilder_block('close');
      mask Display: plot(0, 0, 100, 100,[2, 2, 32, 32, 2], [68, 8, 8, 68, 68],[32, 2], [38, 38], [32, 19, 2],[53, 60, 44], [32, 17, 17, 2],[16, 16, 31, 31]);txt = getActiveGroup(gcbh);text(2, 100, txt,'verticalAlignment', 'top');
  T_env : Outport
  RH_env : Outport  Port=2
  mdot : Outport  Port=3
  S_blend : Outport  Port=4
  S_AC : Outport  Port=5
  S_flap : Outport  Port=6
  wires:
  Signal Builder/2(RH_env) -> RH_env/1
  Fan/1 -> mdot/1
  Heat/1 -> S_blend/1
  AC/1 -> S_AC/1
  Recirculation/1 -> S_flap/1
  Mux/1 -> Scope/1
  [T_vent] -> Mux/2
  [RH_cabin] -> Mux1/3
  [RH_vent] -> Mux1/2
  [RH_env] -> Mux1/1
  [T_cabin] -> Mux/3
  [T_env] -> Mux/1
  Mux1/1 -> Scope/2
  Signal Builder/1(T_env) -> T_env/1

== system vehicleHVAC/System Inputs/Predefined ==
  Signal Builder : Subsystem  Tag=STV Subsys  LoadFcn=sigbuilder_block('load');  StartFcn=sigbuilder_block('start');  StopFcn=sigbuilder_block('stop');  ClipboardFcn=sigbuilder_block('clipboard');  mask(Sigbuilder block){}
      mask help: Simulink:masks:SigbuilderBlock_MD
      mask init:
      | if ~strcmp(get_param(bdroot(gcbh),'SimulationStatus'),'stopped') tuvar = sigbuilder_block('maskInit'); end
      settings: CopyFcn=sigbuilder_block('copy');  DeleteFcn=sigbuilder_block('delete');  ModelCloseFcn=sigbuilder_block('modelClose');  PreSaveFcn=sigbuilder_block('preSave');  PauseFcn=sigbuilder_block('pause');  ContinueFcn=sigbuilder_block('continue');  NameChangeFcn=sigbuilder_block('namechange');  OpenFcn=sigbuilder_block('open',[183 321.75 550.5 504.75 ]);  CloseFcn=sigbuilder_block('close');
      mask Display: plot(0, 0, 100, 100,[2, 2, 32, 32, 2], [68, 8, 8, 68, 68],[32, 2], [38, 38], [32, 19, 2],[53, 60, 44], [32, 17, 17, 2],[16, 16, 31, 31]);txt = getActiveGroup(gcbh);text(2, 100, txt,'verticalAlignment', 'top');
  T_env : Outport
  RH_env : Outport  Port=2
  mdot : Outport  Port=3
  S_blend : Outport  Port=4
  S_AC : Outport  Port=5
  S_flap : Outport  Port=6
  wires:
  Signal Builder/1(T_env) -> T_env/1
  Signal Builder/2(RH_env) -> RH_env/1
  Signal Builder/3(mdot) -> mdot/1
  Signal Builder/4(S_blend) -> S_blend/1
  Signal Builder/6(S_flap) -> S_flap/1
  Signal Builder/5(S_AC) -> S_AC/1

== system vehicleHVAC/System Inputs/Manual/AC Switch ==

== system vehicleHVAC/System Inputs/Manual/Cabin Relative Humidity ==

== system vehicleHVAC/System Inputs/Manual/Cabin Temperature (degC) ==

== system vehicleHVAC/System Inputs/Manual/Fan Dial ==

== system vehicleHVAC/System Inputs/Manual/Heat Dial ==

== system vehicleHVAC/System Inputs/Manual/Recirculation Switch ==

== system vehicleHVAC/System Inputs/Manual/Signal Builder ==
  Demux : Demux  Tag=STV Demux  Outputs=2
  FromWs : FromWorkspace  Tag=STV FromWs  VariableName=tuvar  SampleTime=0
      SigBuilderData=|
      | common.afterFinalStr = 'Extrapolate'
      | common.sampleTime = 0
      | dataSet.timeRange = [0 2000]
      | dataSet.name = 'Group 1'
      | sbobj.Groups.Name = 'Group 1'
      | sbobj.Groups.Signals(1).Name = 'T_env'
      | sbobj.Groups.Signals(1).XData = [0 2000]
      | sbobj.Groups.Signals(1).YData = [25 25]
      | sbobj.Groups.Signals(2).Name = 'RH_env'
      | sbobj.Groups.Signals(2).XData = [0 2000]
      | sbobj.Groups.Signals(2).YData = [0.5 0.5]
      | sbobj.Groups.TimeRange = [0 2000]
  T_env : Outport  Tag=STV Outport
  RH_env : Outport  Tag=STV Outport  Port=2
  wires:
  Demux/1 -> T_env/1
  FromWs/1 -> Demux/1
  Demux/2 -> RH_env/1

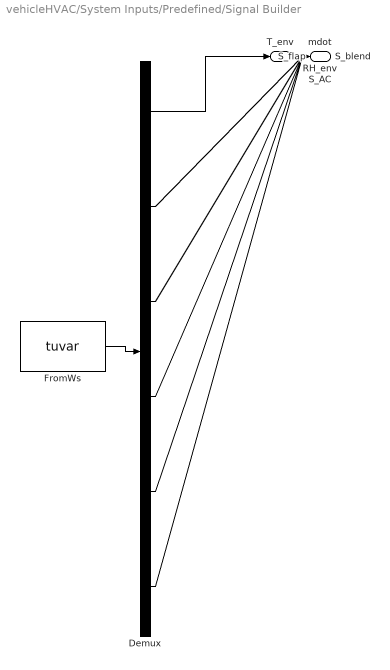
== system vehicleHVAC/System Inputs/Predefined/Signal Builder ==
  Demux : Demux  Tag=STV Demux  Outputs=6
  FromWs : FromWorkspace  Tag=STV FromWs  VariableName=tuvar  SampleTime=0
      SigBuilderData=|
      | common.afterFinalStr = 'Extrapolate'
      | common.sampleTime = '0'
      | dataSet.timeRange = [0 2000]
      | dataSet.name = 'Group 1'
      | sbobj.Groups.Name = 'Group 1'
      | sbobj.Groups.Signals(1).Name = 'T_env'
      | sbobj.Groups.Signals(1).XData = [0 2000]
      | sbobj.Groups.Signals(1).YData = [25 25]
      | sbobj.Groups.Signals(2).Name = 'RH_env'
      | sbobj.Groups.Signals(2).XData = [0 2000]
      | sbobj.Groups.Signals(2).YData = [0.5 0.5]
      | sbobj.Groups.Signals(3).Name = 'mdot'
      | sbobj.Groups.Signals(3).XData = [0 100 100 2000]
      | sbobj.Groups.Signals(3).YData = [0 0 0.06 0.06]
      | sbobj.Groups.Signals(4).Name = 'S_blend'
      | sbobj.Groups.Signals(4).XData = [0 1500 1500 2000]
      | sbobj.Groups.Signals(4).YData = [0 0 0.2 0.2]
      | sbobj.Groups.Signals(5).Name = 'S_AC'
      | sbobj.Groups.Signals(5).XData = [0 300 300 2000]
      | sbobj.Groups.Signals(5).YData = [0 0 1 1]
      | sbobj.Groups.Signals(6).Name = 'S_flap'
      | sbobj.Groups.Signals(6).XData = [0 300 300 1000 1000 2000]
      | sbobj.Groups.Signals(6).YData = [0 0 1 1 0 0]
      | sbobj.Groups.TimeRange = [0 2000]
  T_env : Outport  Tag=STV Outport
  RH_env : Outport  Tag=STV Outport  Port=2
  mdot : Outport  Tag=STV Outport  Port=3
  S_blend : Outport  Tag=STV Outport  Port=4
  S_AC : Outport  Tag=STV Outport  Port=5
  S_flap : Outport  Tag=STV Outport  Port=6
  wires:
  Demux/1 -> T_env/1
  FromWs/1 -> Demux/1
  Demux/2 -> RH_env/1
  Demux/3 -> mdot/1
  Demux/4 -> S_blend/1
  Demux/5 -> S_AC/1
  Demux/6 -> S_flap/1
